simulink model "fgc"  (R2023a)
settings: Solver=ode3  StartTime=0.0  StopTime=inf  FixedStep=0.05  RelTol=1e-3
model workspace (MAT data in the model file):
  set_speed = 1.5
undefined symbols (not defined in the file): Drive
libraries: robotlib x9
settings Model: Creator=pmodi  LastModifiedBy=gptp
settings OptimizationCC: EnhancedBackFolding=on  PassReuseOutputArgsAs=Individual arguments  ZeroExternalMemoryAtStartup=off  ZeroInternalMemoryAtStartup=off  MaxStackSize=64  OptimizeBlockOrder=speed  DifferentSizesBufferReuse=on  OptimizationCustomize=off  EfficientTunableParamExpr=on
settings DebuggingCC: ParameterTunabilityLossMsg=error
settings HardwareCC: ProdBitPerLong=64  ProdLargestAtomicInteger=LongLong  ProdLargestAtomicFloat=Double  ProdLongLongMode=on  ProdHWDeviceType=ARM Compatible->ARM 64-bit (LP64)
settings SFSimCC: MATLABDynamicMemAlloc=off
settings RTWCC: Description=Embedded Coder  SystemTargetFile=ert.tlc  HardwareBoard=Robot Operating System (ROS)  TLCOptions="-aInlineSetEventsForThisBaseRateFcn=TLC_FALSE -aSuppressMultiTaskScheduler=TLC_FALSE  -aRateBasedStepFcn=0"  GenCodeOnly=on  TemplateMakefile=ert_default_tmf  Toolchain=Catkin  TargetLang=C++
settings CodeAppCC: ForceParamTrailComments=on  IgnoreCustomStorageClasses=off  OperatorAnnotations=on  SimulinkDataObjDesc=on  SFDataObjDesc=on  InsertBlockDesc=on
settings ERTTargetCC: SupportVariableSizeSignals=on

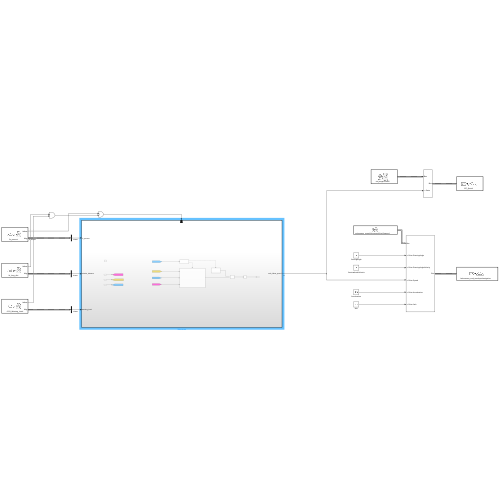
[thumbnail: Simulink's stored preview of the top-level diagram]
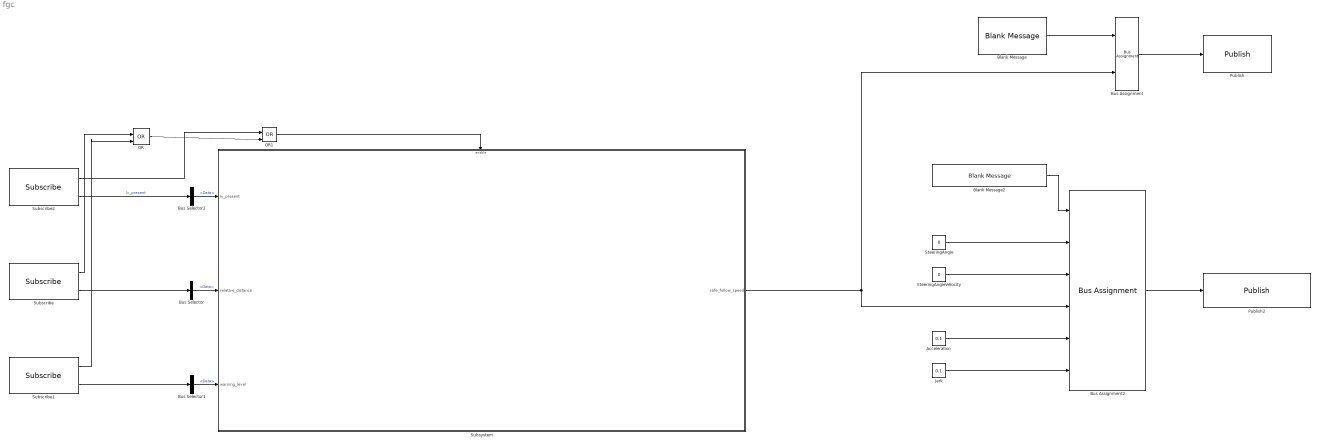
== system fgc ==
  Acceleration : Constant  Value=0.1  OutDataTypeStr=single
  Blank Message : robotlib/Blank Message  messageClass=Message  entityType=std_msgs/Float32  messageType=std_msgs/Float32  SampleTime=inf  legacyBusStruct=off
  Blank Message2 : robotlib/Blank Message  messageClass=Message  entityType=ackermann_msgs/AckermannDriveStamped  messageType=ackermann_msgs/AckermannDriveStamped  SampleTime=inf  legacyBusStruct=off
  Bus Assignment : BusAssignment  AssignedSignals=Data
  Bus Assignment2 : BusAssignment  AssignedSignals=Drive.SteeringAngle,Drive.SteeringAngleVelocity,Drive.Speed,Drive.Acceleration,Drive.Jerk
  Bus Selector : BusSelector  OutputSignals=Data
  Bus Selector1 : BusSelector  OutputSignals=Data
  Bus Selector2 : BusSelector  OutputSignals=Data
  Jerk : Constant  Value=0.1  OutDataTypeStr=single
  OR : Logic  Operator=OR  IconShape=distinctive  AllPortsSameDT=off  OutDataTypeStr=boolean
  OR1 : Logic  Operator=OR  IconShape=distinctive  AllPortsSameDT=off  OutDataTypeStr=boolean
  Publish : robotlib/Publish  topicSource=Specify your own  topic=/SF_Speed  messageType=std_msgs/Float32  legacyBusStruct=off  messageQueueLength=1
  Publish2 : robotlib/Publish  topicSource=Specify your own  topic=/ackermann_cmd_mux/input/navigation  messageType=ackermann_msgs/AckermannDriveStamped  legacyBusStruct=off  messageQueueLength=5
  SteeringAngle : Constant  Value=0  OutDataTypeStr=single
  SteeringAngleVelocity : Constant  Value=0  OutDataTypeStr=single
  Subscribe : robotlib/Subscribe  topicSource=Specify your own  topic=/lv_long_dist  messageType=std_msgs/Float32  SampleTime=-1  legacyBusStruct=off  messageQueueLength=5
  Subscribe1 : robotlib/Subscribe  topicSource=Specify your own  topic=/V2V_Warning_Level  messageType=std_msgs/UInt8  SampleTime=-1  legacyBusStruct=off  messageQueueLength=1
  Subscribe2 : robotlib/Subscribe  topicSource=Specify your own  topic=/lv_present  messageType=std_msgs/Bool  SampleTime=-1  legacyBusStruct=off  messageQueueLength=5
  Subsystem : Subsystem
  wires:
  Bus Assignment2/1 -> Publish2/1
  Bus Assignment/1 -> Publish/1
  Jerk/1 -> Bus Assignment2/6
  SteeringAngleVelocity/1 -> Bus Assignment2/3
  SteeringAngle/1 -> Bus Assignment2/2
  Subscribe/2 -> Bus Selector/1
  Subscribe1/1 -> OR/2
  OR/1 -> OR1/2
  Subscribe/1 -> OR/1
  Subscribe1/2 -> Bus Selector1/1
  Acceleration/1 -> Bus Assignment2/5
  Subscribe2/1 -> OR1/1
  Subscribe2/2 -> Bus Selector2/1  "lv_present"
  Bus Selector/1 -> Subsystem/2(relative_distance)  "<Data>"
  Blank Message2/1 -> Bus Assignment2/1
  Subsystem/1(safe_follow_speed) -> Bus Assignment/2, Bus Assignment2/4
  OR1/1 -> Subsystem/Enable
  Bus Selector2/1 -> Subsystem/1(lv_present)  "<Data>"
  Bus Selector1/1 -> Subsystem/3(warning_level)  "<Data>"
  Blank Message/1 -> Bus Assignment/1

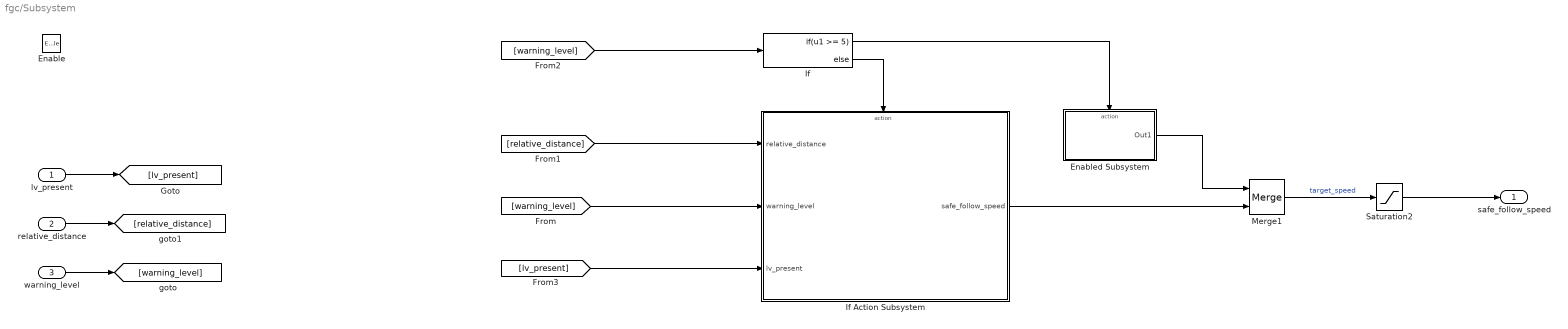
== system fgc/Subsystem ==
  lv_present : Inport
  relative_distance : Inport  Port=2
  warning_level : Inport  Port=3  OutDataTypeStr=uint8
  Enable : EnablePort
  Enabled Subsystem : Subsystem  TreatAsAtomicUnit=on
  If : If  IfExpression=u1 >= 5
  If Action Subsystem : Subsystem  TreatAsAtomicUnit=on
  Merge1 : Merge
  Saturation2 : Saturate  UpperLimit=set_speed  LowerLimit=0
  safe_follow_speed : Outport  OutDataTypeStr=single
  wires:
  [relative_distance] -> If Action Subsystem/1(relative_distance)
  [warning_level] -> If Action Subsystem/2(warning_level)
  relative_distance/1 -> [relative_distance]
  If Action Subsystem/1(safe_follow_speed) -> Merge1/2
  lv_present/1 -> [lv_present]
  warning_level/1 -> [warning_level]
  If/2 -> If Action Subsystem/Action
  If/1 -> Enabled Subsystem/Action
  [warning_level] -> If/1
  Enabled Subsystem/1(Out1) -> Merge1/1
  [lv_present] -> If Action Subsystem/3(lv_present)
  Merge1/1 -> Saturation2/1  "target_speed"
  Saturation2/1 -> safe_follow_speed/1

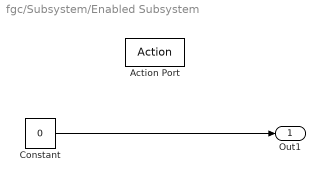
== system fgc/Subsystem/Enabled Subsystem ==
  Action Port : ActionPort  ActionPortLabel=if(u1 >= 5)
  Constant : Constant  Value=0  OutDataTypeStr=single
  Out1 : Outport
  wires:
  Constant/1 -> Out1/1

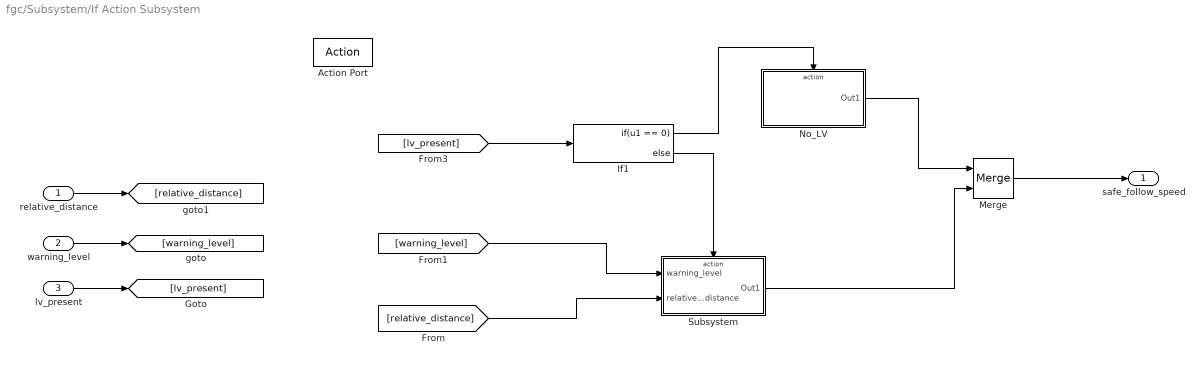
== system fgc/Subsystem/If Action Subsystem ==
  relative_distance : Inport
  warning_level : Inport  Port=2  OutDataTypeStr=uint8
  lv_present : Inport  Port=3
  Action Port : ActionPort  ActionPortLabel=else
  If1 : If  IfExpression=u1 == 0
  Merge : Merge
  No_LV : Subsystem
  Subsystem : Subsystem
  safe_follow_speed : Outport
  wires:
  warning_level/1 -> [warning_level]
  relative_distance/1 -> [relative_distance]
  Merge/1 -> safe_follow_speed/1
  [relative_distance] -> Subsystem/2(relative_distance)
  [warning_level] -> Subsystem/1(warning_level)
  Subsystem/1(Out1) -> Merge/2
  No_LV/1(Out1) -> Merge/1
  [lv_present] -> If1/1
  If1/1 -> No_LV/Action
  If1/2 -> Subsystem/Action
  lv_present/1 -> [lv_present]

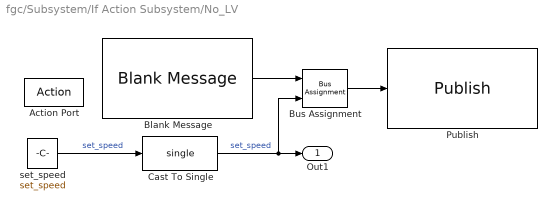
== system fgc/Subsystem/If Action Subsystem/No_LV ==
  Action Port : ActionPort  ActionPortLabel=if(u1 == 0)
  Blank Message : robotlib/Blank Message  messageClass=Message  entityType=std_msgs/Float32  messageType=std_msgs/Float32  SampleTime=inf  legacyBusStruct=off
  Bus Assignment : BusAssignment  AssignedSignals=Data
  Cast To Single : DataTypeConversion  OutDataTypeStr=single  SaturateOnIntegerOverflow=off  RndMeth=Floor
  Publish : robotlib/Publish  topicSource=Specify your own  topic=/debug_sf_speed  messageType=std_msgs/Float32  legacyBusStruct=off  messageQueueLength=1
  set_speed : Constant  Value=set_speed
  Out1 : Outport
  wires:
  Bus Assignment/1 -> Publish/1
  Cast To Single/1 -> Out1/1, Bus Assignment/2  "set_speed"
  Blank Message/1 -> Bus Assignment/1
  set_speed/1 -> Cast To Single/1  "set_speed"

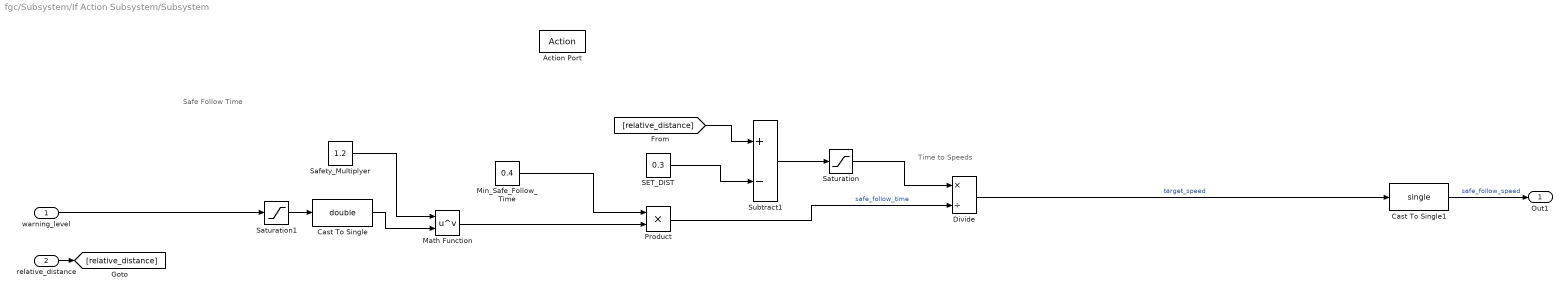
== system fgc/Subsystem/If Action Subsystem/Subsystem ==
  note: Time to Speeds
  note: Safe Follow Time
  warning_level : Inport
  relative_distance : Inport  Port=2
  Action Port : ActionPort  ActionPortLabel=else
  Cast To Single : DataTypeConversion  OutDataTypeStr=double  SaturateOnIntegerOverflow=off  RndMeth=Floor
  Cast To Single1 : DataTypeConversion  OutDataTypeStr=single  SaturateOnIntegerOverflow=off  RndMeth=Floor
  Divide : Product  Inputs=*/
  Math Function : Math  Operator=pow
  Min_Safe_Follow_Time : Constant  Value=0.4
  Product : Product
  SET_DIST : Constant  Value=0.3
  Safety_Multiplyer : Constant  Value=1.2
  Saturation : Saturate  UpperLimit=inf  LowerLimit=0
  Saturation1 : Saturate  UpperLimit=5  LowerLimit=0
  Subtract1 : Sum  Inputs=+-
  Out1 : Outport
  wires:
  warning_level/1 -> Saturation1/1
  Saturation/1 -> Divide/1
  Saturation1/1 -> Cast To Single/1
  Product/1 -> Divide/2  "safe_follow_time"
  Subtract1/1 -> Saturation/1
  SET_DIST/1 -> Subtract1/2
  Cast To Single/1 -> Math Function/2
  [relative_distance] -> Subtract1/1
  Min_Safe_Follow_Time/1 -> Product/1
  Math Function/1 -> Product/2
  Safety_Multiplyer/1 -> Math Function/1
  Cast To Single1/1 -> Out1/1  "safe_follow_speed"
  relative_distance/1 -> [relative_distance]
  Divide/1 -> Cast To Single1/1  "target_speed"
